simulink model "nonlinear_LQR"  (R2021b)
settings: Solver=VariableStepAuto  StartTime=0.0  StopTime=100  RelTol=1e-3
settings Model: Creator=Anubhav Paras  LastModifiedBy=vanshika
settings SolverCC: AlgebraicLoopSolver=TrustRegion
settings DebuggingCC: SFMachineParentedDataDiag=warning

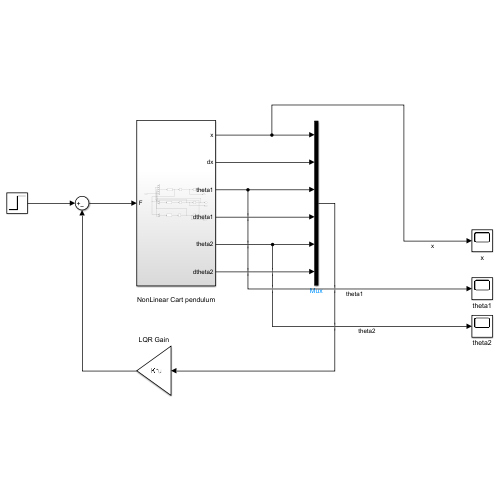
[thumbnail: Simulink's stored preview of the top-level diagram]
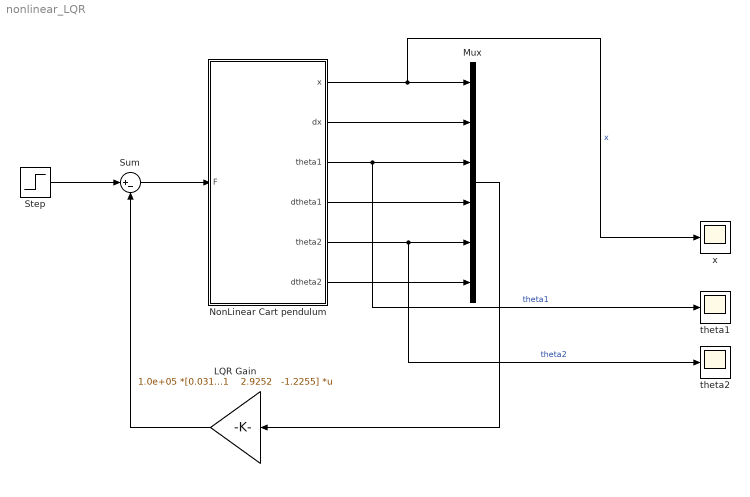
== system nonlinear_LQR ==
  " NonLinear Cart pendulum" : Subsystem
  LQR Gain : Gain  Gain="1.0e+05 *[0.0316    0.1518    0.6176    1.1011    2.9252   -1.2255]"  Multiplication=Matrix(K*u)
  Mux : Mux  Inputs=6
  Step : Step  SampleTime=100
  Sum : Sum  Inputs=|+-
  theta1 : Scope
  theta2 : Scope
  x : Scope
  wires:
  " NonLinear Cart pendulum"/1(x) -> Mux/1, x/1  "x"
  " NonLinear Cart pendulum"/2(dx) -> Mux/2
  " NonLinear Cart pendulum"/3(theta1) -> Mux/3, theta1/1  "theta1"
  " NonLinear Cart pendulum"/4(dtheta1) -> Mux/4
  " NonLinear Cart pendulum"/5(theta2) -> Mux/5, theta2/1  "theta2"
  " NonLinear Cart pendulum"/6(dtheta2) -> Mux/6
  Mux/1 -> LQR Gain/1
  Step/1 -> Sum/1
  Sum/1 -> " NonLinear Cart pendulum"/1(F)
  LQR Gain/1 -> Sum/2

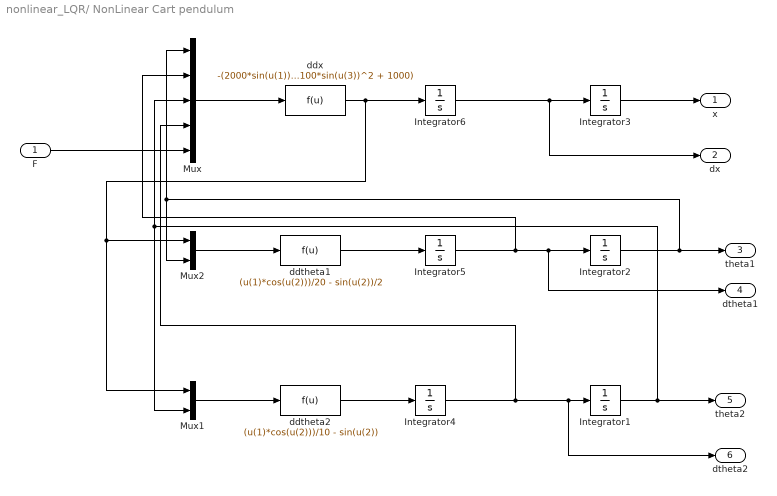
== system nonlinear_LQR/ NonLinear Cart pendulum ==
  F : Inport
  Integrator1 : Integrator  InitialCondition=0.1
  Integrator2 : Integrator  InitialCondition=0.1
  Integrator3 : Integrator  InitialCondition=0.5
  Integrator4 : Integrator
  Integrator5 : Integrator
  Integrator6 : Integrator
  Mux : Mux  Inputs=5
  Mux1 : Mux  Inputs=2
  Mux2 : Mux  Inputs=2
  ddtheta1 : Fcn  Expr=(u(1)*cos(u(2)))/20 - sin(u(2))/2
  ddtheta2 : Fcn  Expr=(u(1)*cos(u(2)))/10 - sin(u(2))
  ddx : Fcn  Expr=-(2000*sin(u(1))*u(2)^2 + 1000*sin(u(3))*u(4)^2 - u(5) + 1000*cos(u(1))*sin(u(1)) - 1000*cos(u(3))*sin(u(3)))/(100*sin(u(1))^2 + 100*sin(u(3))^2 + 1000)
  x : Outport
  dx : Outport  Port=2
  theta1 : Outport  Port=3
  dtheta1 : Outport  Port=4
  theta2 : Outport  Port=5
  dtheta2 : Outport  Port=6
  wires:
  ddtheta2/1 -> Integrator4/1
  ddx/1 -> Mux1/1, Mux2/1, Integrator6/1
  Integrator6/1 -> Integrator3/1, dx/1
  Mux1/1 -> ddtheta2/1
  Integrator5/1 -> Mux/2, Integrator2/1, dtheta1/1
  Mux/1 -> ddx/1
  Integrator1/1 -> theta2/1, Mux1/2, Mux/3
  Integrator2/1 -> theta1/1, Mux2/2, Mux/1
  ddtheta1/1 -> Integrator5/1
  Integrator4/1 -> Mux/4, Integrator1/1, dtheta2/1
  Mux2/1 -> ddtheta1/1
  Integrator3/1 -> x/1
  F/1 -> Mux/5
